simulink model "RL_analog"  (R2020a)
settings: Solver=ode45  StartTime=0.0  StopTime=0.005  MaxStep=1e-6  RelTol=1e-3
values from neighbouring files (symbols this model uses):
  d = [-1/Ld; 0]    [sim_set_RL_Load_analog.m]
  J = skewdec(2,0)    [sim_set_RL_Load_analog.m]
  ki = wn^2*Ld    (= 393061.22449)    [sim_set_RL_Load_analog.m]
  kp = 2*xi*wn*Ld-R    (= 127.8)    [sim_set_RL_Load_analog.m]
  Ld = 21.4e-3    (= 0.0214)    [sim_set_RL_Load_analog.m]
  Linv = inv(L)    [sim_set_RL_Load_analog.m]
  Lq = 21.4e-3    (= 0.0214)    [sim_set_RL_Load_analog.m]
  p = 5    [sim_set_RL_Load_analog.m]
  Rs = R    (= 0.6)    [sim_set_RL_Load_analog.m]
  wm = 2*pi*50    (= 314.159265359)    [sim_set_RL_Load_analog.m]
settings Model: Creator=Nicky  LastModifiedBy=Nicky

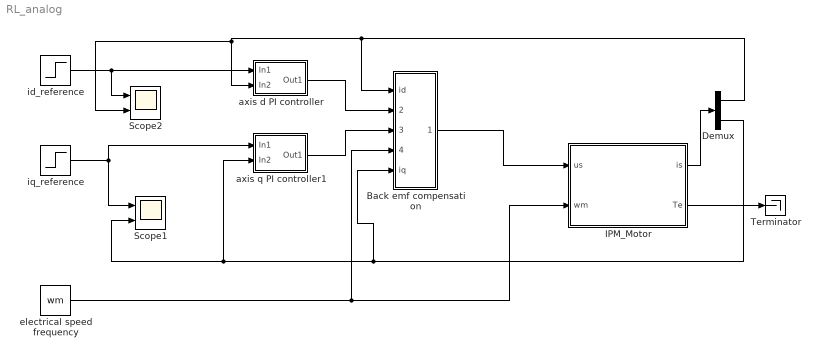
== system RL_analog ==
  Back emf compensation : Subsystem
  Demux : Demux  Outputs=2
  IPM_Motor : Subsystem
  Scope1 : Scope  NumInputPorts=2
  Scope2 : Scope  NumInputPorts=2
  Terminator : Terminator
  axis d PI controller : Subsystem
  axis q PI controller1 : Subsystem
  electrical speed frequency : Constant  Value=wm
  id_reference : Step  Time=0.001  After=0.5  SampleTime=0
  iq_reference : Step  Time=0.0025  After=-0.5  SampleTime=0
  wires:
  electrical speed frequency/1 -> IPM_Motor/2(wm), Back emf compensation/4(In3)
  id_reference/1 -> Scope2/1, axis d PI controller/1(In1)
  iq_reference/1 -> Scope1/1, axis q PI controller1/1(In1)
  IPM_Motor/2(Te) -> Terminator/1
  axis d PI controller/1(Out1) -> Back emf compensation/2(In1)
  axis q PI controller1/1(Out1) -> Back emf compensation/3(In2)
  Back emf compensation/1(Out1) -> IPM_Motor/1(us)
  IPM_Motor/1(is) -> Demux/1
  Demux/1 -> Back emf compensation/1(id), Scope2/2, axis d PI controller/2(In2)
  Demux/2 -> Back emf compensation/5(iq), axis q PI controller1/2(In2), Scope1/2

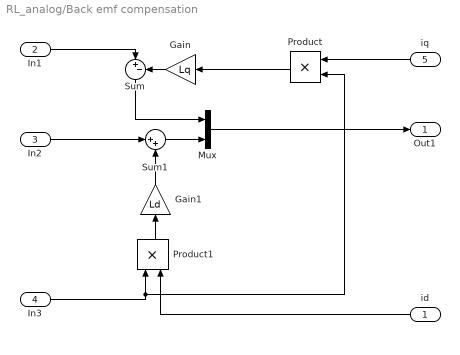
== system RL_analog/Back emf compensation ==
  id : Inport
  In1 : Inport  Port=2
  In2 : Inport  Port=3
  In3 : Inport  Port=4
  iq : Inport  Port=5
  Gain : Gain  Gain=Lq
  Gain1 : Gain  Gain=Ld
  Mux : Mux  Inputs=2
  Product : Product
  Product1 : Product
  Sum : Sum  Inputs=|+-
  Sum1 : Sum  Inputs=|++
  Out1 : Outport
  wires:
  In1/1 -> Sum/1
  Gain1/1 -> Sum1/2
  Mux/1 -> Out1/1
  Sum1/1 -> Mux/2
  Gain/1 -> Sum/2
  Sum/1 -> Mux/1
  In2/1 -> Sum1/1
  iq/1 -> Product/1
  Product/1 -> Gain/1
  In3/1 -> Product/2, Product1/1
  Product1/1 -> Gain1/1
  id/1 -> Product1/2

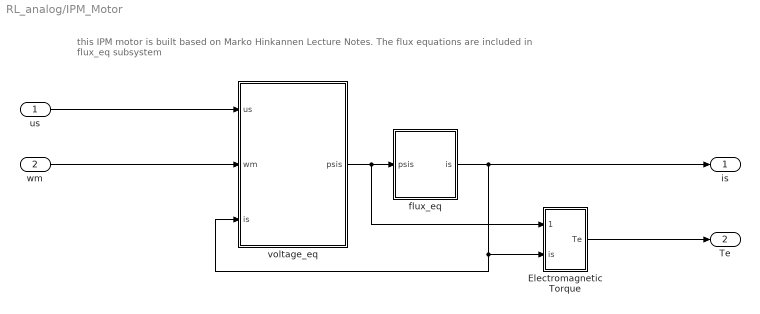
== system RL_analog/IPM_Motor ==
  note: this IPM motor is built based on Marko Hinkannen Lecture Notes. The flux equations are included in flux_eq subsystem
  us : Inport
  wm : Inport  Port=2
  Electromagnetic Torque : Subsystem
  flux_eq : Subsystem
  voltage_eq : Subsystem
  is : Outport  VectorParamsAs1DForOutWhenUnconnected=off
  Te : Outport  Port=2  VectorParamsAs1DForOutWhenUnconnected=off
  wires:
  wm/1 -> voltage_eq/2(wm)
  us/1 -> voltage_eq/1(us)
  flux_eq/1(is) -> is/1, Electromagnetic Torque/2(is), voltage_eq/3(is)
  voltage_eq/1(psis) -> Electromagnetic Torque/1(psis), flux_eq/1(psis)
  Electromagnetic Torque/1(Te) -> Te/1

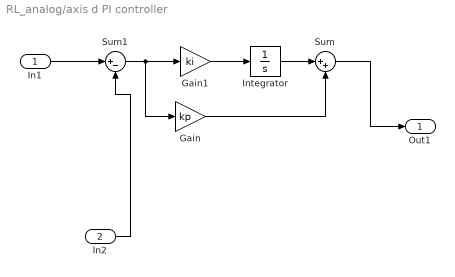
== system RL_analog/axis d PI controller ==
  In1 : Inport
  In2 : Inport  Port=2
  Gain : Gain  Gain=kp
  Gain1 : Gain  Gain=ki
  Integrator : Integrator
  Sum : Sum  Inputs=|++
  Sum1 : Sum  Inputs=|+-
  Out1 : Outport
  wires:
  In1/1 -> Sum1/1
  Sum/1 -> Out1/1
  Gain/1 -> Sum/2
  Sum1/1 -> Gain1/1, Gain/1
  Gain1/1 -> Integrator/1
  In2/1 -> Sum1/2
  Integrator/1 -> Sum/1

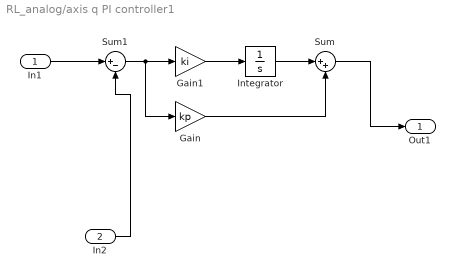
== system RL_analog/axis q PI controller1 ==
  In1 : Inport
  In2 : Inport  Port=2
  Gain : Gain  Gain=kp
  Gain1 : Gain  Gain=ki
  Integrator : Integrator
  Sum : Sum  Inputs=|++
  Sum1 : Sum  Inputs=|+-
  Out1 : Outport
  wires:
  In1/1 -> Sum1/1
  Sum/1 -> Out1/1
  Gain/1 -> Sum/2
  Sum1/1 -> Gain1/1, Gain/1
  Gain1/1 -> Integrator/1
  In2/1 -> Sum1/2
  Integrator/1 -> Sum/1

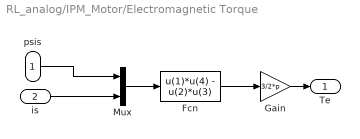
== system RL_analog/IPM_Motor/Electromagnetic Torque ==
  psis : Inport
  is : Inport  Port=2
  Fcn : Fcn  Expr=u(1)*u(4) - u(2)*u(3)
  Gain : Gain  Gain=3/2*p
  Mux : Mux  Inputs=2
  Te : Outport  VectorParamsAs1DForOutWhenUnconnected=off
  wires:
  Gain/1 -> Te/1
  is/1 -> Mux/2
  psis/1 -> Mux/1
  Mux/1 -> Fcn/1
  Fcn/1 -> Gain/1

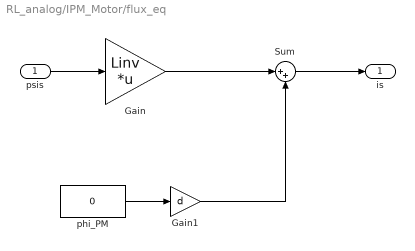
== system RL_analog/IPM_Motor/flux_eq ==
  psis : Inport
  Gain : Gain  Gain=Linv  Multiplication=Matrix(K*u) (u vector)
  Gain1 : Gain  Gain=d
  Sum : Sum  Inputs=|++
  phi_PM : Constant  Value=0
  is : Outport  VectorParamsAs1DForOutWhenUnconnected=off
  wires:
  psis/1 -> Gain/1
  phi_PM/1 -> Gain1/1
  Gain/1 -> Sum/1
  Gain1/1 -> Sum/2
  Sum/1 -> is/1

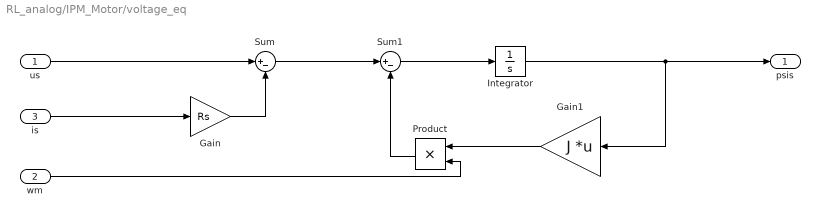
== system RL_analog/IPM_Motor/voltage_eq ==
  us : Inport
  wm : Inport  Port=2
  is : Inport  Port=3
  Gain : Gain  Gain=Rs
  Gain1 : Gain  Gain=J  Multiplication=Matrix(K*u) (u vector)
  Integrator : Integrator
  Product : Product
  Sum : Sum  Inputs=|+-
  Sum1 : Sum  Inputs=|+-
  psis : Outport  VectorParamsAs1DForOutWhenUnconnected=off
  wires:
  Integrator/1 -> Gain1/1, psis/1
  Gain/1 -> Sum/2
  Sum1/1 -> Integrator/1
  us/1 -> Sum/1
  wm/1 -> Product/2
  Product/1 -> Sum1/2
  is/1 -> Gain/1
  Sum/1 -> Sum1/1
  Gain1/1 -> Product/1
